simulink model "batterpack"  (R2024b)
settings: Solver=VariableStepAuto  StartTime=0.0  StopTime=10.0  RelTol=1e-3
libraries: spsParallelRLCBranchLib x432, spsDCVoltageSourceLib x144, spsIdealSwitchLib x14, spsTriangleGeneratorLib x1, spspowerguiLib x1
settings Model: Creator=32635  LastModifiedBy=32635

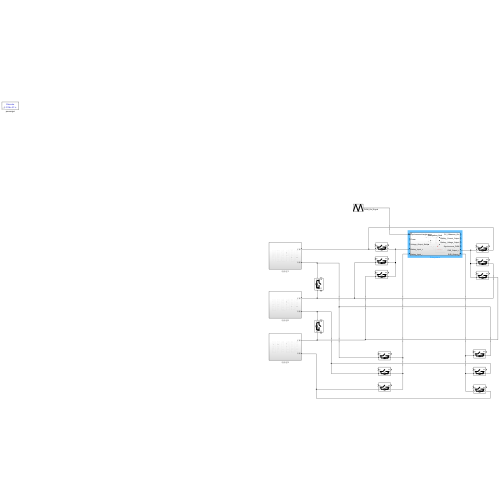
[thumbnail: Simulink's stored preview of the top-level diagram]
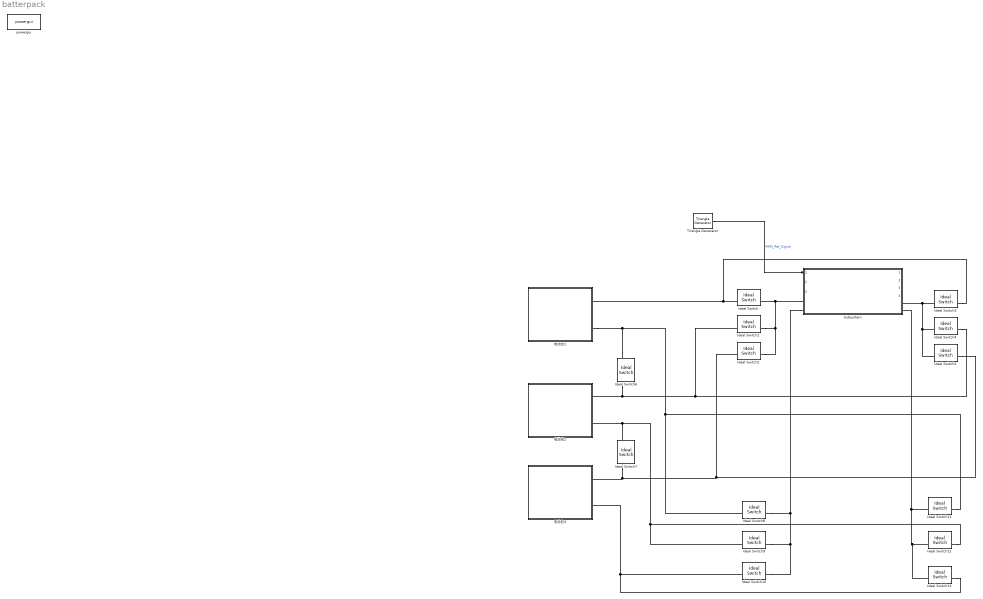
== system batterpack ==
  Ideal Switch{,1..13} (14 alike) : spsIdealSwitchLib/Ideal Switch  Ron=0.001  Lon=0  IC=0  Rs=1e5  Cs=inf  Measurements=on
  Subsystem : Subsystem  ReferencedSubsystem=Subsystem_final
  Triangle Generator : spsTriangleGeneratorLib/Triangle Generator  Freq=50000  Phase=0  Ts=0
  powergui : spspowerguiLib/powergui  Priority=1  SimulationMode=Discrete  SampleTime=1/5e4/60  frequency=60  Iterations=50  frequencyindice=0  Pbase=100e6  ErrMax=1e-4  UnitsV=kV  UnitsW=MW  buscounter=0  FunctionMessages=off  echomessages=off  EnableUseOfTLC=off  CurrentSourceSwitches=off  DisableSnubberDevices=off  DisableRonSwitches=off  DisableVfSwitches=off  DisplayEquations=off  AutomaticDiscreteSolvers=off  SolverType=Tustin/Backward Euler (TBE)  Interpol=off  ExternalGateDelay=off  methode=off  Ts=100  x0status=blocks  SPID=on  SwTol=0  HookPort=off  NonlinearTolerance=1e-4  nMaxIteration=100  ContinueOnMaxIteration=off  RestoreLinks=warning  ResistiveCurrentMeasurement=off  Frange=[0:2:500]  Ylog=off  Xlog=on  ShowGrid=off  save=off  variable=ZData  structure=0  ZoomFFT=on  StartTime=0.0  cycles=1  DisplayStyle=1  fundamental=60  FreqAxis=off  MaxFrequency=1000  frequencyindicesteady=1  RmsSteady=1  display=off
  电池包1 : Subsystem
  电池包2 : Subsystem
  电池包3 : Subsystem
  wires:
  Triangle Generator/1 -> Subsystem/1  "PWM_Ref_Signal"
  connections:
  Ideal Switch2/LConn1 -- Ideal Switch5/RConn1 -- 电池包3/RConn1 -- Ideal Switch7/RConn1
  Ideal Switch1/LConn1 -- Ideal Switch4/RConn1 -- Ideal Switch6/RConn1 -- 电池包2/RConn1
  Subsystem/LConn1 -- Ideal Switch2/RConn1 -- Ideal Switch1/RConn1 -- Ideal Switch/RConn1
  Ideal Switch/LConn1 -- Ideal Switch3/RConn1 -- 电池包1/RConn1
  Ideal Switch7/LConn1 -- Ideal Switch12/RConn1 -- Ideal Switch9/LConn1 -- 电池包2/RConn2
  Ideal Switch3/LConn1 -- Ideal Switch4/LConn1 -- Ideal Switch5/LConn1 -- Subsystem/RConn1
  电池包1/RConn2 -- Ideal Switch11/RConn1 -- Ideal Switch8/LConn1 -- Ideal Switch6/LConn1
  Ideal Switch8/RConn1 -- Ideal Switch10/RConn1 -- Ideal Switch9/RConn1 -- Subsystem/LConn2
  Ideal Switch10/LConn1 -- 电池包3/RConn2 -- Ideal Switch13/RConn1
  Ideal Switch11/LConn1 -- Ideal Switch13/LConn1 -- Ideal Switch12/LConn1 -- Subsystem/RConn2

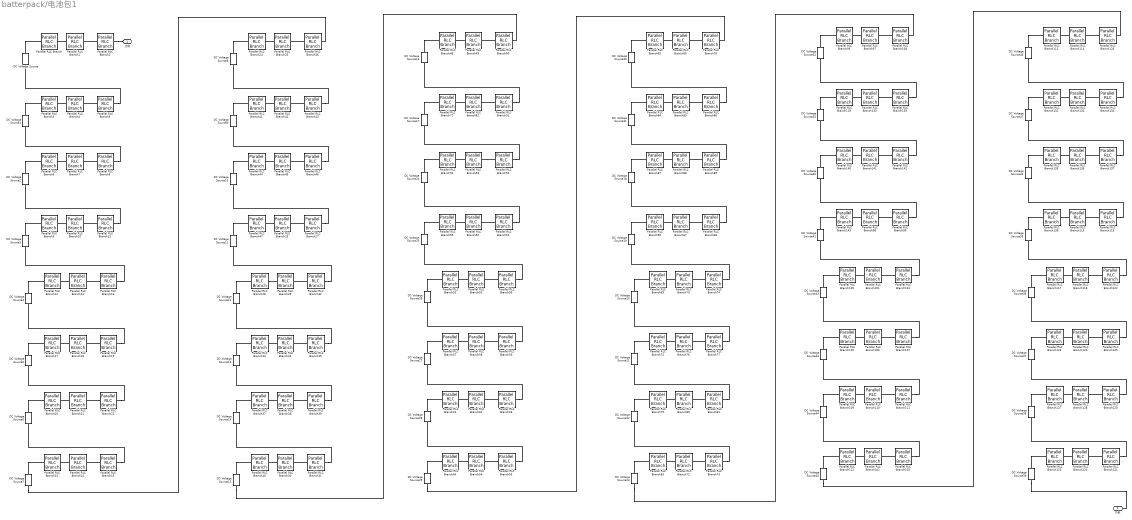
== system batterpack/电池包1 ==
  DC Voltage Source{,1..47} (48 alike) : spsDCVoltageSourceLib/DC Voltage Source  Amplitude=100  Measurements=None
  Parallel RLC Branch{,3,6,9,12,17,20,23..24,28,33,37,40..41,44,47..48,52,57,61,64..65,69,71,75,79,83..84,87,90,92,95..96,100,105,109,112..113,117,119,123,127,131..132,135,138,140,143} (48 alike) : spsParallelRLCBranchLib/Parallel RLC Branch  LConnTagsString=a  RConnTagsString=__new0  BranchType=R  Resistance=1  Inductance=1e-3  SetiL0=off  InitialCurrent=0  Capacitance=1e-6  Setx0=off  InitialVoltage=0  Measurements=None
  Parallel RLC Branch{1..2,4..5,7..8,10..11,13..16,18..19,21..22,25..27,29..32,34..36,38..39,42..43,45..46,49..51,53..56,58..60,62..63,66..68,70,72..74,76..78,80..82,85..86,88..89,91,93..94,97..99,101..104,106..108,110..111,114..116,118,120..122,124..126,128..130,133..134,136..137,139,141..142} (96 alike) : spsParallelRLCBranchLib/Parallel RLC Branch  LConnTagsString=a  RConnTagsString=__new0  BranchType=RC  Resistance=1  Inductance=1e-3  SetiL0=off  InitialCurrent=0  Capacitance=1e-6  Setx0=off  InitialVoltage=0  Measurements=None
  正极 : PMIOPort  Side=Right
  负极 : PMIOPort  Port=2  Side=Right
  connections:
  Parallel RLC Branch81/RConn1 -- DC Voltage Source21/LConn1
  Parallel RLC Branch48/LConn1 -- DC Voltage Source16/RConn1
  Parallel RLC Branch1/LConn1 -- Parallel RLC Branch/RConn1
  Parallel RLC Branch45/LConn1 -- Parallel RLC Branch44/RConn1
  Parallel RLC Branch129/RConn1 -- DC Voltage Source37/LConn1
  Parallel RLC Branch143/LConn1 -- DC Voltage Source41/RConn1
  Parallel RLC Branch8/RConn1 -- DC Voltage Source1/LConn1
  Parallel RLC Branch133/LConn1 -- Parallel RLC Branch132/RConn1
  Parallel RLC Branch87/LConn1 -- DC Voltage Source18/RConn1
  Parallel RLC Branch86/RConn1 -- DC Voltage Source30/LConn1
  Parallel RLC Branch123/LConn1 -- DC Voltage Source37/RConn1
  Parallel RLC Branch32/LConn1 -- Parallel RLC Branch29/RConn1
  Parallel RLC Branch44/LConn1 -- DC Voltage Source10/RConn1
  Parallel RLC Branch10/LConn1 -- Parallel RLC Branch9/RConn1
  DC Voltage Source15/LConn1 -- Parallel RLC Branch60/RConn1
  Parallel RLC Branch4/LConn1 -- Parallel RLC Branch3/RConn1
  Parallel RLC Branch74/RConn1 -- DC Voltage Source19/LConn1
  Parallel RLC Branch24/LConn1 -- DC Voltage Source8/RConn1
  Parallel RLC Branch107/RConn1 -- DC Voltage Source42/LConn1
  Parallel RLC Branch139/RConn1 -- DC Voltage Source32/LConn1
  Parallel RLC Branch39/LConn1 -- Parallel RLC Branch38/RConn1
  Parallel RLC Branch137/LConn1 -- Parallel RLC Branch136/RConn1
  Parallel RLC Branch126/LConn1 -- Parallel RLC Branch114/RConn1
  Parallel RLC Branch91/RConn1 -- DC Voltage Source16/LConn1
  DC Voltage Source29/LConn1 -- Parallel RLC Branch78/RConn1
  Parallel RLC Branch42/LConn1 -- Parallel RLC Branch41/RConn1
  Parallel RLC Branch68/RConn1 -- DC Voltage Source18/LConn1
  Parallel RLC Branch136/LConn1 -- Parallel RLC Branch135/RConn1
  Parallel RLC Branch5/RConn1 -- DC Voltage Source/LConn1
  Parallel RLC Branch55/LConn1 -- Parallel RLC Branch54/RConn1
  Parallel RLC Branch22/LConn1 -- Parallel RLC Branch21/RConn1
  Parallel RLC Branch27/LConn1 -- Parallel RLC Branch26/RConn1
  DC Voltage Source23/LConn1 -- Parallel RLC Branch108/RConn1
  Parallel RLC Branch80/LConn1 -- Parallel RLC Branch79/RConn1
  Parallel RLC Branch41/LConn1 -- DC Voltage Source9/RConn1
  DC Voltage Source7/LConn1 -- Parallel RLC Branch36/RConn1
  Parallel RLC Branch139/LConn1 -- Parallel RLC Branch130/RConn1
  Parallel RLC Branch99/LConn1 -- Parallel RLC Branch98/RConn1
  Parallel RLC Branch56/LConn1 -- Parallel RLC Branch53/RConn1
  Parallel RLC Branch113/LConn1 -- DC Voltage Source46/RConn1
  Parallel RLC Branch103/RConn1 -- DC Voltage Source44/LConn1
  Parallel RLC Branch94/LConn1 -- Parallel RLC Branch93/RConn1
  Parallel RLC Branch81/LConn1 -- Parallel RLC Branch80/RConn1
  Parallel RLC Branch140/LConn1 -- DC Voltage Source40/RConn1
  Parallel RLC Branch60/LConn1 -- Parallel RLC Branch49/RConn1
  Parallel RLC Branch63/LConn1 -- Parallel RLC Branch62/RConn1
  Parallel RLC Branch29/LConn1 -- Parallel RLC Branch28/RConn1
  Parallel RLC Branch104/RConn1 -- DC Voltage Source41/LConn1
  Parallel RLC Branch142/RConn1 -- DC Voltage Source33/LConn1
  Parallel RLC Branch2/LConn1 -- Parallel RLC Branch1/RConn1
  Parallel RLC Branch114/LConn1 -- Parallel RLC Branch113/RConn1
  Parallel RLC Branch16/RConn1 -- DC Voltage Source3/LConn1
  Parallel RLC Branch116/LConn1 -- Parallel RLC Branch115/RConn1
  Parallel RLC Branch67/LConn1 -- Parallel RLC Branch90/RConn1
  Parallel RLC Branch51/LConn1 -- Parallel RLC Branch50/RConn1
  Parallel RLC Branch46/LConn1 -- Parallel RLC Branch45/RConn1
  Parallel RLC Branch121/LConn1 -- Parallel RLC Branch120/RConn1
  Parallel RLC Branch104/LConn1 -- Parallel RLC Branch101/RConn1
  Parallel RLC Branch85/LConn1 -- Parallel RLC Branch84/RConn1
  Parallel RLC Branch99/RConn1 -- DC Voltage Source40/LConn1
  Parallel RLC Branch53/LConn1 -- Parallel RLC Branch52/RConn1
  Parallel RLC Branch101/LConn1 -- Parallel RLC Branch100/RConn1
  Parallel RLC Branch47/LConn1 -- DC Voltage Source11/RConn1
  Parallel RLC Branch103/LConn1 -- Parallel RLC Branch102/RConn1
  Parallel RLC Branch125/RConn1 -- DC Voltage Source36/LConn1
  Parallel RLC Branch61/LConn1 -- DC Voltage Source28/RConn1
  Parallel RLC Branch91/LConn1 -- Parallel RLC Branch82/RConn1
  Parallel RLC Branch26/LConn1 -- Parallel RLC Branch47/RConn1
  Parallel RLC Branch124/LConn1 -- Parallel RLC Branch123/RConn1
  Parallel RLC Branch132/LConn1 -- DC Voltage Source47/RConn1
  Parallel RLC Branch64/LConn1 -- DC Voltage Source29/RConn1
  Parallel RLC Branch50/LConn1 -- Parallel RLC Branch95/RConn1
  Parallel RLC Branch35/LConn1 -- Parallel RLC Branch34/RConn1
  Parallel RLC Branch30/LConn1 -- Parallel RLC Branch40/RConn1
  Parallel RLC Branch28/LConn1 -- DC Voltage Source12/RConn1
  Parallel RLC Branch86/LConn1 -- Parallel RLC Branch85/RConn1
  Parallel RLC Branch57/LConn1 -- DC Voltage Source27/RConn1
  Parallel RLC Branch13/LConn1 -- Parallel RLC Branch12/RConn1
  Parallel RLC Branch58/LConn1 -- Parallel RLC Branch57/RConn1
  Parallel RLC Branch37/LConn1 -- DC Voltage Source14/RConn1
  Parallel RLC Branch63/RConn1 -- DC Voltage Source27/LConn1
  Parallel RLC Branch/LConn1 -- DC Voltage Source/RConn1
  Parallel RLC Branch73/LConn1 -- Parallel RLC Branch72/RConn1
  Parallel RLC Branch54/LConn1 -- Parallel RLC Branch64/RConn1
  Parallel RLC Branch77/LConn1 -- Parallel RLC Branch76/RConn1
  Parallel RLC Branch76/LConn1 -- Parallel RLC Branch75/RConn1
  Parallel RLC Branch73/RConn1 -- DC Voltage Source22/LConn1
  Parallel RLC Branch31/RConn1 -- DC Voltage Source14/LConn1
  Parallel RLC Branch112/LConn1 -- DC Voltage Source45/RConn1
  Parallel RLC Branch70/LConn1 -- Parallel RLC Branch69/RConn1
  Parallel RLC Branch15/LConn1 -- Parallel RLC Branch14/RConn1
  Parallel RLC Branch59/LConn1 -- Parallel RLC Branch58/RConn1
  Parallel RLC Branch35/RConn1 -- DC Voltage Source12/LConn1
  Parallel RLC Branch49/LConn1 -- Parallel RLC Branch48/RConn1
  Parallel RLC Branch69/LConn1 -- DC Voltage Source20/RConn1
  Parallel RLC Branch51/RConn1 -- DC Voltage Source24/LConn1
  Parallel RLC Branch134/RConn1 -- DC Voltage Source46/LConn1
  Parallel RLC Branch72/LConn1 -- Parallel RLC Branch83/RConn1
  Parallel RLC Branch55/RConn1 -- DC Voltage Source28/LConn1
  Parallel RLC Branch84/LConn1 -- DC Voltage Source31/RConn1
  Parallel RLC Branch78/LConn1 -- Parallel RLC Branch66/RConn1
  Parallel RLC Branch15/RConn1 -- DC Voltage Source6/LConn1
  Parallel RLC Branch83/LConn1 -- DC Voltage Source23/RConn1
  Parallel RLC Branch117/LConn1 -- DC Voltage Source36/RConn1
  Parallel RLC Branch74/LConn1 -- Parallel RLC Branch70/RConn1
  Parallel RLC Branch90/LConn1 -- DC Voltage Source19/RConn1
  Parallel RLC Branch89/LConn1 -- Parallel RLC Branch88/RConn1
  Parallel RLC Branch106/LConn1 -- Parallel RLC Branch105/RConn1
  Parallel RLC Branch62/LConn1 -- Parallel RLC Branch61/RConn1
  Parallel RLC Branch52/LConn1 -- DC Voltage Source26/RConn1
  Parallel RLC Branch88/LConn1 -- Parallel RLC Branch87/RConn1
  Parallel RLC Branch129/LConn1 -- Parallel RLC Branch128/RConn1
  Parallel RLC Branch96/LConn1 -- DC Voltage Source32/RConn1
  Parallel RLC Branch94/RConn1 -- DC Voltage Source17/LConn1
  Parallel RLC Branch95/LConn1 -- DC Voltage Source25/RConn1
  Parallel RLC Branch56/RConn1 -- DC Voltage Source25/LConn1
  Parallel RLC Branch92/LConn1 -- DC Voltage Source24/RConn1
  Parallel RLC Branch75/LConn1 -- DC Voltage Source21/RConn1
  Parallel RLC Branch89/RConn1 -- DC Voltage Source31/LConn1
  Parallel RLC Branch111/LConn1 -- Parallel RLC Branch110/RConn1
  Parallel RLC Branch66/LConn1 -- Parallel RLC Branch65/RConn1
  Parallel RLC Branch77/RConn1 -- DC Voltage Source20/LConn1
  Parallel RLC Branch68/LConn1 -- Parallel RLC Branch67/RConn1
  Parallel RLC Branch120/LConn1 -- Parallel RLC Branch131/RConn1
  DC Voltage Source45/LConn1 -- Parallel RLC Branch126/RConn1
  Parallel RLC Branch97/LConn1 -- Parallel RLC Branch96/RConn1
  Parallel RLC Branch36/LConn1 -- Parallel RLC Branch25/RConn1
  Parallel RLC Branch9/LConn1 -- DC Voltage Source3/RConn1
  Parallel RLC Branch93/LConn1 -- Parallel RLC Branch92/RConn1
  Parallel RLC Branch79/LConn1 -- DC Voltage Source22/RConn1
  Parallel RLC Branch65/LConn1 -- DC Voltage Source30/RConn1
  Parallel RLC Branch71/LConn1 -- DC Voltage Source17/RConn1
  Parallel RLC Branch82/LConn1 -- Parallel RLC Branch71/RConn1
  Parallel RLC Branch59/RConn1 -- DC Voltage Source26/LConn1
  Parallel RLC Branch22/RConn1 -- DC Voltage Source5/LConn1
  Parallel RLC Branch18/LConn1 -- Parallel RLC Branch17/RConn1
  Parallel RLC Branch20/LConn1 -- DC Voltage Source6/RConn1
  Parallel RLC Branch12/LConn1 -- DC Voltage Source4/RConn1
  Parallel RLC Branch19/RConn1 -- DC Voltage Source4/LConn1
  Parallel RLC Branch16/LConn1 -- Parallel RLC Branch13/RConn1
  Parallel RLC Branch23/LConn1 -- DC Voltage Source7/RConn1
  Parallel RLC Branch19/LConn1 -- Parallel RLC Branch18/RConn1
  Parallel RLC Branch14/LConn1 -- Parallel RLC Branch23/RConn1
  Parallel RLC Branch17/LConn1 -- DC Voltage Source5/RConn1
  Parallel RLC Branch138/LConn1 -- DC Voltage Source35/RConn1
  Parallel RLC Branch21/LConn1 -- Parallel RLC Branch20/RConn1
  Parallel RLC Branch25/LConn1 -- Parallel RLC Branch24/RConn1
  Parallel RLC Branch27/RConn1 -- DC Voltage Source10/LConn1
  Parallel RLC Branch33/LConn1 -- DC Voltage Source13/RConn1
  Parallel RLC Branch32/RConn1 -- DC Voltage Source11/LConn1
  Parallel RLC Branch108/LConn1 -- Parallel RLC Branch97/RConn1
  Parallel RLC Branch34/LConn1 -- Parallel RLC Branch33/RConn1
  Parallel RLC Branch43/RConn1 -- DC Voltage Source8/LConn1
  Parallel RLC Branch31/LConn1 -- Parallel RLC Branch30/RConn1
  Parallel RLC Branch46/RConn1 -- DC Voltage Source9/LConn1
  Parallel RLC Branch40/LConn1 -- DC Voltage Source15/RConn1
  Parallel RLC Branch39/RConn1 -- DC Voltage Source13/LConn1
  Parallel RLC Branch135/LConn1 -- DC Voltage Source34/RConn1
  Parallel RLC Branch110/LConn1 -- Parallel RLC Branch109/RConn1
  Parallel RLC Branch100/LConn1 -- DC Voltage Source42/RConn1
  Parallel RLC Branch43/LConn1 -- Parallel RLC Branch42/RConn1
  Parallel RLC Branch5/LConn1 -- Parallel RLC Branch4/RConn1
  Parallel RLC Branch3/LConn1 -- DC Voltage Source1/RConn1
  Parallel RLC Branch6/LConn1 -- DC Voltage Source2/RConn1
  Parallel RLC Branch11/LConn1 -- Parallel RLC Branch10/RConn1
  Parallel RLC Branch107/LConn1 -- Parallel RLC Branch106/RConn1
  Parallel RLC Branch8/LConn1 -- Parallel RLC Branch7/RConn1
  Parallel RLC Branch11/RConn1 -- DC Voltage Source2/LConn1
  Parallel RLC Branch118/LConn1 -- Parallel RLC Branch117/RConn1
  Parallel RLC Branch7/LConn1 -- Parallel RLC Branch6/RConn1
  Parallel RLC Branch38/LConn1 -- Parallel RLC Branch37/RConn1
  Parallel RLC Branch134/LConn1 -- Parallel RLC Branch133/RConn1
  Parallel RLC Branch119/LConn1 -- DC Voltage Source33/RConn1
  Parallel RLC Branch142/LConn1 -- Parallel RLC Branch141/RConn1
  Parallel RLC Branch130/LConn1 -- Parallel RLC Branch119/RConn1
  Parallel RLC Branch131/LConn1 -- DC Voltage Source39/RConn1
  Parallel RLC Branch105/LConn1 -- DC Voltage Source43/RConn1
  Parallel RLC Branch127/LConn1 -- DC Voltage Source38/RConn1
  Parallel RLC Branch122/LConn1 -- Parallel RLC Branch118/RConn1
  Parallel RLC Branch116/RConn1 -- DC Voltage Source34/LConn1
  Parallel RLC Branch122/RConn1 -- DC Voltage Source35/LConn1
  Parallel RLC Branch98/LConn1 -- Parallel RLC Branch143/RConn1
  Parallel RLC Branch128/LConn1 -- Parallel RLC Branch127/RConn1
  Parallel RLC Branch115/LConn1 -- Parallel RLC Branch138/RConn1
  Parallel RLC Branch121/RConn1 -- DC Voltage Source38/LConn1
  Parallel RLC Branch109/LConn1 -- DC Voltage Source44/RConn1
  Parallel RLC Branch141/LConn1 -- Parallel RLC Branch140/RConn1
  Parallel RLC Branch137/RConn1 -- DC Voltage Source47/LConn1
  Parallel RLC Branch102/LConn1 -- Parallel RLC Branch112/RConn1
  Parallel RLC Branch111/RConn1 -- DC Voltage Source43/LConn1
  Parallel RLC Branch125/LConn1 -- Parallel RLC Branch124/RConn1
  DC Voltage Source39/LConn1 -- 负极/RConn1
  Parallel RLC Branch2/RConn1 -- 正极/RConn1

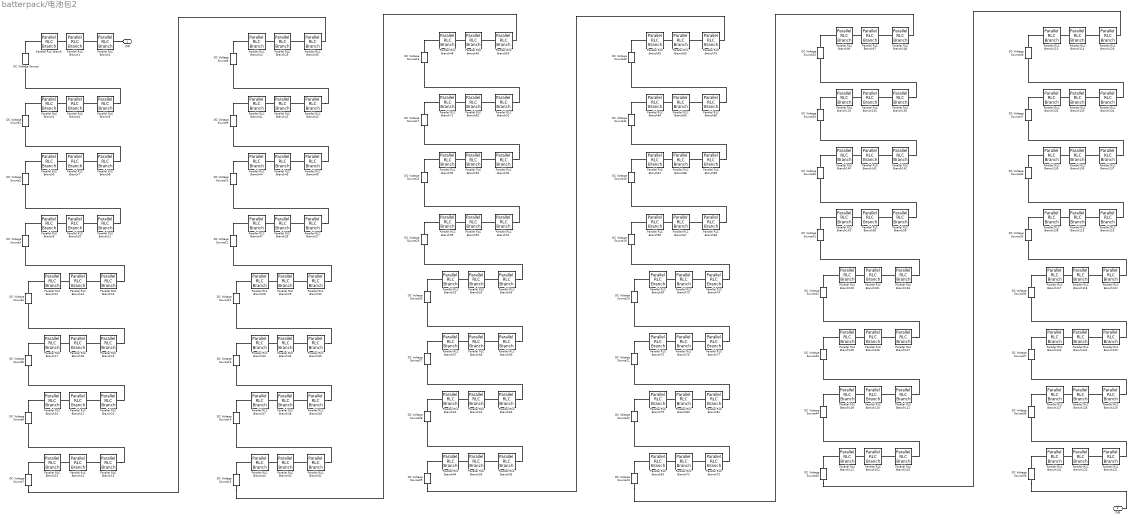
== system batterpack/电池包2 ==
  DC Voltage Source{,1..47} (48 alike) : spsDCVoltageSourceLib/DC Voltage Source  Amplitude=100  Measurements=None
  Parallel RLC Branch{,3,6,9,12,17,20,23..24,28,33,37,40..41,44,47..48,52,57,61,64..65,69,71,75,79,83..84,87,90,92,95..96,100,105,109,112..113,117,119,123,127,131..132,135,138,140,143} (48 alike) : spsParallelRLCBranchLib/Parallel RLC Branch  LConnTagsString=a  RConnTagsString=__new0  BranchType=R  Resistance=1  Inductance=1e-3  SetiL0=off  InitialCurrent=0  Capacitance=1e-6  Setx0=off  InitialVoltage=0  Measurements=None
  Parallel RLC Branch{1..2,4..5,7..8,10..11,13..16,18..19,21..22,25..27,29..32,34..36,38..39,42..43,45..46,49..51,53..56,58..60,62..63,66..68,70,72..74,76..78,80..82,85..86,88..89,91,93..94,97..99,101..104,106..108,110..111,114..116,118,120..122,124..126,128..130,133..134,136..137,139,141..142} (96 alike) : spsParallelRLCBranchLib/Parallel RLC Branch  LConnTagsString=a  RConnTagsString=__new0  BranchType=RC  Resistance=1  Inductance=1e-3  SetiL0=off  InitialCurrent=0  Capacitance=1e-6  Setx0=off  InitialVoltage=0  Measurements=None
  正极 : PMIOPort  Side=Right
  负极 : PMIOPort  Port=2  Side=Right
  connections:
  Parallel RLC Branch2/RConn1 -- 正极/RConn1
  DC Voltage Source39/LConn1 -- 负极/RConn1
  Parallel RLC Branch125/LConn1 -- Parallel RLC Branch124/RConn1
  Parallel RLC Branch111/RConn1 -- DC Voltage Source43/LConn1
  Parallel RLC Branch102/LConn1 -- Parallel RLC Branch112/RConn1
  Parallel RLC Branch137/RConn1 -- DC Voltage Source47/LConn1
  Parallel RLC Branch141/LConn1 -- Parallel RLC Branch140/RConn1
  Parallel RLC Branch109/LConn1 -- DC Voltage Source44/RConn1
  Parallel RLC Branch121/RConn1 -- DC Voltage Source38/LConn1
  Parallel RLC Branch115/LConn1 -- Parallel RLC Branch138/RConn1
  Parallel RLC Branch128/LConn1 -- Parallel RLC Branch127/RConn1
  Parallel RLC Branch98/LConn1 -- Parallel RLC Branch143/RConn1
  Parallel RLC Branch122/RConn1 -- DC Voltage Source35/LConn1
  Parallel RLC Branch116/RConn1 -- DC Voltage Source34/LConn1
  Parallel RLC Branch122/LConn1 -- Parallel RLC Branch118/RConn1
  Parallel RLC Branch127/LConn1 -- DC Voltage Source38/RConn1
  Parallel RLC Branch105/LConn1 -- DC Voltage Source43/RConn1
  Parallel RLC Branch131/LConn1 -- DC Voltage Source39/RConn1
  Parallel RLC Branch130/LConn1 -- Parallel RLC Branch119/RConn1
  Parallel RLC Branch142/LConn1 -- Parallel RLC Branch141/RConn1
  Parallel RLC Branch119/LConn1 -- DC Voltage Source33/RConn1
  Parallel RLC Branch134/LConn1 -- Parallel RLC Branch133/RConn1
  Parallel RLC Branch38/LConn1 -- Parallel RLC Branch37/RConn1
  Parallel RLC Branch7/LConn1 -- Parallel RLC Branch6/RConn1
  Parallel RLC Branch118/LConn1 -- Parallel RLC Branch117/RConn1
  Parallel RLC Branch11/RConn1 -- DC Voltage Source2/LConn1
  Parallel RLC Branch8/LConn1 -- Parallel RLC Branch7/RConn1
  Parallel RLC Branch107/LConn1 -- Parallel RLC Branch106/RConn1
  Parallel RLC Branch11/LConn1 -- Parallel RLC Branch10/RConn1
  Parallel RLC Branch6/LConn1 -- DC Voltage Source2/RConn1
  Parallel RLC Branch3/LConn1 -- DC Voltage Source1/RConn1
  Parallel RLC Branch5/LConn1 -- Parallel RLC Branch4/RConn1
  Parallel RLC Branch43/LConn1 -- Parallel RLC Branch42/RConn1
  Parallel RLC Branch100/LConn1 -- DC Voltage Source42/RConn1
  Parallel RLC Branch110/LConn1 -- Parallel RLC Branch109/RConn1
  Parallel RLC Branch135/LConn1 -- DC Voltage Source34/RConn1
  Parallel RLC Branch39/RConn1 -- DC Voltage Source13/LConn1
  Parallel RLC Branch40/LConn1 -- DC Voltage Source15/RConn1
  Parallel RLC Branch46/RConn1 -- DC Voltage Source9/LConn1
  Parallel RLC Branch31/LConn1 -- Parallel RLC Branch30/RConn1
  Parallel RLC Branch43/RConn1 -- DC Voltage Source8/LConn1
  Parallel RLC Branch34/LConn1 -- Parallel RLC Branch33/RConn1
  Parallel RLC Branch108/LConn1 -- Parallel RLC Branch97/RConn1
  Parallel RLC Branch32/RConn1 -- DC Voltage Source11/LConn1
  Parallel RLC Branch33/LConn1 -- DC Voltage Source13/RConn1
  Parallel RLC Branch27/RConn1 -- DC Voltage Source10/LConn1
  Parallel RLC Branch25/LConn1 -- Parallel RLC Branch24/RConn1
  Parallel RLC Branch21/LConn1 -- Parallel RLC Branch20/RConn1
  Parallel RLC Branch138/LConn1 -- DC Voltage Source35/RConn1
  Parallel RLC Branch17/LConn1 -- DC Voltage Source5/RConn1
  Parallel RLC Branch14/LConn1 -- Parallel RLC Branch23/RConn1
  Parallel RLC Branch19/LConn1 -- Parallel RLC Branch18/RConn1
  Parallel RLC Branch23/LConn1 -- DC Voltage Source7/RConn1
  Parallel RLC Branch16/LConn1 -- Parallel RLC Branch13/RConn1
  Parallel RLC Branch19/RConn1 -- DC Voltage Source4/LConn1
  Parallel RLC Branch12/LConn1 -- DC Voltage Source4/RConn1
  Parallel RLC Branch20/LConn1 -- DC Voltage Source6/RConn1
  Parallel RLC Branch18/LConn1 -- Parallel RLC Branch17/RConn1
  Parallel RLC Branch22/RConn1 -- DC Voltage Source5/LConn1
  Parallel RLC Branch59/RConn1 -- DC Voltage Source26/LConn1
  Parallel RLC Branch82/LConn1 -- Parallel RLC Branch71/RConn1
  Parallel RLC Branch71/LConn1 -- DC Voltage Source17/RConn1
  Parallel RLC Branch65/LConn1 -- DC Voltage Source30/RConn1
  Parallel RLC Branch79/LConn1 -- DC Voltage Source22/RConn1
  Parallel RLC Branch93/LConn1 -- Parallel RLC Branch92/RConn1
  Parallel RLC Branch9/LConn1 -- DC Voltage Source3/RConn1
  Parallel RLC Branch36/LConn1 -- Parallel RLC Branch25/RConn1
  Parallel RLC Branch97/LConn1 -- Parallel RLC Branch96/RConn1
  DC Voltage Source45/LConn1 -- Parallel RLC Branch126/RConn1
  Parallel RLC Branch120/LConn1 -- Parallel RLC Branch131/RConn1
  Parallel RLC Branch68/LConn1 -- Parallel RLC Branch67/RConn1
  Parallel RLC Branch77/RConn1 -- DC Voltage Source20/LConn1
  Parallel RLC Branch66/LConn1 -- Parallel RLC Branch65/RConn1
  Parallel RLC Branch111/LConn1 -- Parallel RLC Branch110/RConn1
  Parallel RLC Branch89/RConn1 -- DC Voltage Source31/LConn1
  Parallel RLC Branch75/LConn1 -- DC Voltage Source21/RConn1
  Parallel RLC Branch92/LConn1 -- DC Voltage Source24/RConn1
  Parallel RLC Branch56/RConn1 -- DC Voltage Source25/LConn1
  Parallel RLC Branch95/LConn1 -- DC Voltage Source25/RConn1
  Parallel RLC Branch94/RConn1 -- DC Voltage Source17/LConn1
  Parallel RLC Branch96/LConn1 -- DC Voltage Source32/RConn1
  Parallel RLC Branch129/LConn1 -- Parallel RLC Branch128/RConn1
  Parallel RLC Branch88/LConn1 -- Parallel RLC Branch87/RConn1
  Parallel RLC Branch52/LConn1 -- DC Voltage Source26/RConn1
  Parallel RLC Branch62/LConn1 -- Parallel RLC Branch61/RConn1
  Parallel RLC Branch106/LConn1 -- Parallel RLC Branch105/RConn1
  Parallel RLC Branch89/LConn1 -- Parallel RLC Branch88/RConn1
  Parallel RLC Branch90/LConn1 -- DC Voltage Source19/RConn1
  Parallel RLC Branch74/LConn1 -- Parallel RLC Branch70/RConn1
  Parallel RLC Branch117/LConn1 -- DC Voltage Source36/RConn1
  Parallel RLC Branch83/LConn1 -- DC Voltage Source23/RConn1
  Parallel RLC Branch15/RConn1 -- DC Voltage Source6/LConn1
  Parallel RLC Branch78/LConn1 -- Parallel RLC Branch66/RConn1
  Parallel RLC Branch84/LConn1 -- DC Voltage Source31/RConn1
  Parallel RLC Branch55/RConn1 -- DC Voltage Source28/LConn1
  Parallel RLC Branch72/LConn1 -- Parallel RLC Branch83/RConn1
  Parallel RLC Branch134/RConn1 -- DC Voltage Source46/LConn1
  Parallel RLC Branch51/RConn1 -- DC Voltage Source24/LConn1
  Parallel RLC Branch69/LConn1 -- DC Voltage Source20/RConn1
  Parallel RLC Branch49/LConn1 -- Parallel RLC Branch48/RConn1
  Parallel RLC Branch35/RConn1 -- DC Voltage Source12/LConn1
  Parallel RLC Branch59/LConn1 -- Parallel RLC Branch58/RConn1
  Parallel RLC Branch15/LConn1 -- Parallel RLC Branch14/RConn1
  Parallel RLC Branch70/LConn1 -- Parallel RLC Branch69/RConn1
  Parallel RLC Branch112/LConn1 -- DC Voltage Source45/RConn1
  Parallel RLC Branch31/RConn1 -- DC Voltage Source14/LConn1
  Parallel RLC Branch73/RConn1 -- DC Voltage Source22/LConn1
  Parallel RLC Branch76/LConn1 -- Parallel RLC Branch75/RConn1
  Parallel RLC Branch77/LConn1 -- Parallel RLC Branch76/RConn1
  Parallel RLC Branch54/LConn1 -- Parallel RLC Branch64/RConn1
  Parallel RLC Branch73/LConn1 -- Parallel RLC Branch72/RConn1
  Parallel RLC Branch/LConn1 -- DC Voltage Source/RConn1
  Parallel RLC Branch63/RConn1 -- DC Voltage Source27/LConn1
  Parallel RLC Branch37/LConn1 -- DC Voltage Source14/RConn1
  Parallel RLC Branch58/LConn1 -- Parallel RLC Branch57/RConn1
  Parallel RLC Branch13/LConn1 -- Parallel RLC Branch12/RConn1
  Parallel RLC Branch57/LConn1 -- DC Voltage Source27/RConn1
  Parallel RLC Branch86/LConn1 -- Parallel RLC Branch85/RConn1
  Parallel RLC Branch28/LConn1 -- DC Voltage Source12/RConn1
  Parallel RLC Branch30/LConn1 -- Parallel RLC Branch40/RConn1
  Parallel RLC Branch35/LConn1 -- Parallel RLC Branch34/RConn1
  Parallel RLC Branch50/LConn1 -- Parallel RLC Branch95/RConn1
  Parallel RLC Branch64/LConn1 -- DC Voltage Source29/RConn1
  Parallel RLC Branch132/LConn1 -- DC Voltage Source47/RConn1
  Parallel RLC Branch124/LConn1 -- Parallel RLC Branch123/RConn1
  Parallel RLC Branch26/LConn1 -- Parallel RLC Branch47/RConn1
  Parallel RLC Branch91/LConn1 -- Parallel RLC Branch82/RConn1
  Parallel RLC Branch61/LConn1 -- DC Voltage Source28/RConn1
  Parallel RLC Branch125/RConn1 -- DC Voltage Source36/LConn1
  Parallel RLC Branch103/LConn1 -- Parallel RLC Branch102/RConn1
  Parallel RLC Branch47/LConn1 -- DC Voltage Source11/RConn1
  Parallel RLC Branch101/LConn1 -- Parallel RLC Branch100/RConn1
  Parallel RLC Branch53/LConn1 -- Parallel RLC Branch52/RConn1
  Parallel RLC Branch99/RConn1 -- DC Voltage Source40/LConn1
  Parallel RLC Branch85/LConn1 -- Parallel RLC Branch84/RConn1
  Parallel RLC Branch104/LConn1 -- Parallel RLC Branch101/RConn1
  Parallel RLC Branch121/LConn1 -- Parallel RLC Branch120/RConn1
  Parallel RLC Branch46/LConn1 -- Parallel RLC Branch45/RConn1
  Parallel RLC Branch51/LConn1 -- Parallel RLC Branch50/RConn1
  Parallel RLC Branch67/LConn1 -- Parallel RLC Branch90/RConn1
  Parallel RLC Branch116/LConn1 -- Parallel RLC Branch115/RConn1
  Parallel RLC Branch16/RConn1 -- DC Voltage Source3/LConn1
  Parallel RLC Branch114/LConn1 -- Parallel RLC Branch113/RConn1
  Parallel RLC Branch2/LConn1 -- Parallel RLC Branch1/RConn1
  Parallel RLC Branch142/RConn1 -- DC Voltage Source33/LConn1
  Parallel RLC Branch104/RConn1 -- DC Voltage Source41/LConn1
  Parallel RLC Branch29/LConn1 -- Parallel RLC Branch28/RConn1
  Parallel RLC Branch63/LConn1 -- Parallel RLC Branch62/RConn1
  Parallel RLC Branch60/LConn1 -- Parallel RLC Branch49/RConn1
  Parallel RLC Branch140/LConn1 -- DC Voltage Source40/RConn1
  Parallel RLC Branch81/LConn1 -- Parallel RLC Branch80/RConn1
  Parallel RLC Branch94/LConn1 -- Parallel RLC Branch93/RConn1
  Parallel RLC Branch103/RConn1 -- DC Voltage Source44/LConn1
  Parallel RLC Branch113/LConn1 -- DC Voltage Source46/RConn1
  Parallel RLC Branch56/LConn1 -- Parallel RLC Branch53/RConn1
  Parallel RLC Branch99/LConn1 -- Parallel RLC Branch98/RConn1
  Parallel RLC Branch139/LConn1 -- Parallel RLC Branch130/RConn1
  DC Voltage Source7/LConn1 -- Parallel RLC Branch36/RConn1
  Parallel RLC Branch41/LConn1 -- DC Voltage Source9/RConn1
  Parallel RLC Branch80/LConn1 -- Parallel RLC Branch79/RConn1
  DC Voltage Source23/LConn1 -- Parallel RLC Branch108/RConn1
  Parallel RLC Branch27/LConn1 -- Parallel RLC Branch26/RConn1
  Parallel RLC Branch22/LConn1 -- Parallel RLC Branch21/RConn1
  Parallel RLC Branch55/LConn1 -- Parallel RLC Branch54/RConn1
  Parallel RLC Branch5/RConn1 -- DC Voltage Source/LConn1
  Parallel RLC Branch136/LConn1 -- Parallel RLC Branch135/RConn1
  Parallel RLC Branch68/RConn1 -- DC Voltage Source18/LConn1
  Parallel RLC Branch42/LConn1 -- Parallel RLC Branch41/RConn1
  DC Voltage Source29/LConn1 -- Parallel RLC Branch78/RConn1
  Parallel RLC Branch91/RConn1 -- DC Voltage Source16/LConn1
  Parallel RLC Branch126/LConn1 -- Parallel RLC Branch114/RConn1
  Parallel RLC Branch137/LConn1 -- Parallel RLC Branch136/RConn1
  Parallel RLC Branch39/LConn1 -- Parallel RLC Branch38/RConn1
  Parallel RLC Branch139/RConn1 -- DC Voltage Source32/LConn1
  Parallel RLC Branch107/RConn1 -- DC Voltage Source42/LConn1
  Parallel RLC Branch24/LConn1 -- DC Voltage Source8/RConn1
  Parallel RLC Branch74/RConn1 -- DC Voltage Source19/LConn1
  Parallel RLC Branch4/LConn1 -- Parallel RLC Branch3/RConn1
  DC Voltage Source15/LConn1 -- Parallel RLC Branch60/RConn1
  Parallel RLC Branch10/LConn1 -- Parallel RLC Branch9/RConn1
  Parallel RLC Branch44/LConn1 -- DC Voltage Source10/RConn1
  Parallel RLC Branch32/LConn1 -- Parallel RLC Branch29/RConn1
  Parallel RLC Branch123/LConn1 -- DC Voltage Source37/RConn1
  Parallel RLC Branch86/RConn1 -- DC Voltage Source30/LConn1
  Parallel RLC Branch87/LConn1 -- DC Voltage Source18/RConn1
  Parallel RLC Branch133/LConn1 -- Parallel RLC Branch132/RConn1
  Parallel RLC Branch8/RConn1 -- DC Voltage Source1/LConn1
  Parallel RLC Branch143/LConn1 -- DC Voltage Source41/RConn1
  Parallel RLC Branch129/RConn1 -- DC Voltage Source37/LConn1
  Parallel RLC Branch45/LConn1 -- Parallel RLC Branch44/RConn1
  Parallel RLC Branch1/LConn1 -- Parallel RLC Branch/RConn1
  Parallel RLC Branch48/LConn1 -- DC Voltage Source16/RConn1
  Parallel RLC Branch81/RConn1 -- DC Voltage Source21/LConn1

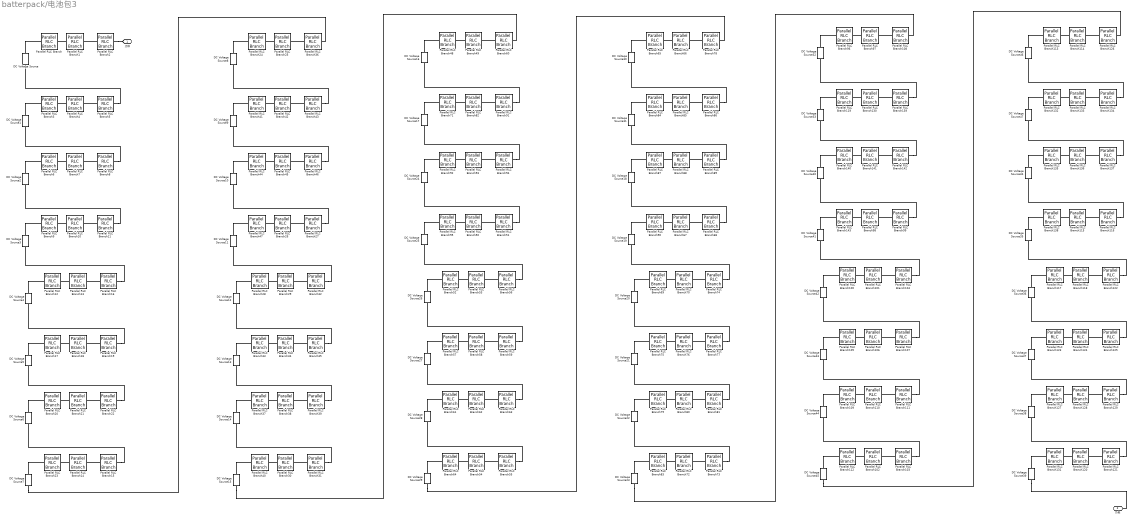
== system batterpack/电池包3 ==
  DC Voltage Source{,1..47} (48 alike) : spsDCVoltageSourceLib/DC Voltage Source  Amplitude=100  Measurements=None
  Parallel RLC Branch{,3,6,9,12,17,20,23..24,28,33,37,40..41,44,47..48,52,57,61,64..65,69,71,75,79,83..84,87,90,92,95..96,100,105,109,112..113,117,119,123,127,131..132,135,138,140,143} (48 alike) : spsParallelRLCBranchLib/Parallel RLC Branch  LConnTagsString=a  RConnTagsString=__new0  BranchType=R  Resistance=1  Inductance=1e-3  SetiL0=off  InitialCurrent=0  Capacitance=1e-6  Setx0=off  InitialVoltage=0  Measurements=None
  Parallel RLC Branch{1..2,4..5,7..8,10..11,13..16,18..19,21..22,25..27,29..32,34..36,38..39,42..43,45..46,49..51,53..56,58..60,62..63,66..68,70,72..74,76..78,80..82,85..86,88..89,91,93..94,97..99,101..104,106..108,110..111,114..116,118,120..122,124..126,128..130,133..134,136..137,139,141..142} (96 alike) : spsParallelRLCBranchLib/Parallel RLC Branch  LConnTagsString=a  RConnTagsString=__new0  BranchType=RC  Resistance=1  Inductance=1e-3  SetiL0=off  InitialCurrent=0  Capacitance=1e-6  Setx0=off  InitialVoltage=0  Measurements=None
  正极 : PMIOPort  Side=Right
  负极 : PMIOPort  Port=2  Side=Right
  connections:
  Parallel RLC Branch81/RConn1 -- DC Voltage Source21/LConn1
  Parallel RLC Branch48/LConn1 -- DC Voltage Source16/RConn1
  Parallel RLC Branch1/LConn1 -- Parallel RLC Branch/RConn1
  Parallel RLC Branch45/LConn1 -- Parallel RLC Branch44/RConn1
  Parallel RLC Branch129/RConn1 -- DC Voltage Source37/LConn1
  Parallel RLC Branch143/LConn1 -- DC Voltage Source41/RConn1
  Parallel RLC Branch8/RConn1 -- DC Voltage Source1/LConn1
  Parallel RLC Branch133/LConn1 -- Parallel RLC Branch132/RConn1
  Parallel RLC Branch87/LConn1 -- DC Voltage Source18/RConn1
  Parallel RLC Branch86/RConn1 -- DC Voltage Source30/LConn1
  Parallel RLC Branch123/LConn1 -- DC Voltage Source37/RConn1
  Parallel RLC Branch32/LConn1 -- Parallel RLC Branch29/RConn1
  Parallel RLC Branch44/LConn1 -- DC Voltage Source10/RConn1
  Parallel RLC Branch10/LConn1 -- Parallel RLC Branch9/RConn1
  DC Voltage Source15/LConn1 -- Parallel RLC Branch60/RConn1
  Parallel RLC Branch4/LConn1 -- Parallel RLC Branch3/RConn1
  Parallel RLC Branch74/RConn1 -- DC Voltage Source19/LConn1
  Parallel RLC Branch24/LConn1 -- DC Voltage Source8/RConn1
  Parallel RLC Branch107/RConn1 -- DC Voltage Source42/LConn1
  Parallel RLC Branch139/RConn1 -- DC Voltage Source32/LConn1
  Parallel RLC Branch39/LConn1 -- Parallel RLC Branch38/RConn1
  Parallel RLC Branch137/LConn1 -- Parallel RLC Branch136/RConn1
  Parallel RLC Branch126/LConn1 -- Parallel RLC Branch114/RConn1
  Parallel RLC Branch91/RConn1 -- DC Voltage Source16/LConn1
  DC Voltage Source29/LConn1 -- Parallel RLC Branch78/RConn1
  Parallel RLC Branch42/LConn1 -- Parallel RLC Branch41/RConn1
  Parallel RLC Branch68/RConn1 -- DC Voltage Source18/LConn1
  Parallel RLC Branch136/LConn1 -- Parallel RLC Branch135/RConn1
  Parallel RLC Branch5/RConn1 -- DC Voltage Source/LConn1
  Parallel RLC Branch55/LConn1 -- Parallel RLC Branch54/RConn1
  Parallel RLC Branch22/LConn1 -- Parallel RLC Branch21/RConn1
  Parallel RLC Branch27/LConn1 -- Parallel RLC Branch26/RConn1
  DC Voltage Source23/LConn1 -- Parallel RLC Branch108/RConn1
  Parallel RLC Branch80/LConn1 -- Parallel RLC Branch79/RConn1
  Parallel RLC Branch41/LConn1 -- DC Voltage Source9/RConn1
  DC Voltage Source7/LConn1 -- Parallel RLC Branch36/RConn1
  Parallel RLC Branch139/LConn1 -- Parallel RLC Branch130/RConn1
  Parallel RLC Branch99/LConn1 -- Parallel RLC Branch98/RConn1
  Parallel RLC Branch56/LConn1 -- Parallel RLC Branch53/RConn1
  Parallel RLC Branch113/LConn1 -- DC Voltage Source46/RConn1
  Parallel RLC Branch103/RConn1 -- DC Voltage Source44/LConn1
  Parallel RLC Branch94/LConn1 -- Parallel RLC Branch93/RConn1
  Parallel RLC Branch81/LConn1 -- Parallel RLC Branch80/RConn1
  Parallel RLC Branch140/LConn1 -- DC Voltage Source40/RConn1
  Parallel RLC Branch60/LConn1 -- Parallel RLC Branch49/RConn1
  Parallel RLC Branch63/LConn1 -- Parallel RLC Branch62/RConn1
  Parallel RLC Branch29/LConn1 -- Parallel RLC Branch28/RConn1
  Parallel RLC Branch104/RConn1 -- DC Voltage Source41/LConn1
  Parallel RLC Branch142/RConn1 -- DC Voltage Source33/LConn1
  Parallel RLC Branch2/LConn1 -- Parallel RLC Branch1/RConn1
  Parallel RLC Branch114/LConn1 -- Parallel RLC Branch113/RConn1
  Parallel RLC Branch16/RConn1 -- DC Voltage Source3/LConn1
  Parallel RLC Branch116/LConn1 -- Parallel RLC Branch115/RConn1
  Parallel RLC Branch67/LConn1 -- Parallel RLC Branch90/RConn1
  Parallel RLC Branch51/LConn1 -- Parallel RLC Branch50/RConn1
  Parallel RLC Branch46/LConn1 -- Parallel RLC Branch45/RConn1
  Parallel RLC Branch121/LConn1 -- Parallel RLC Branch120/RConn1
  Parallel RLC Branch104/LConn1 -- Parallel RLC Branch101/RConn1
  Parallel RLC Branch85/LConn1 -- Parallel RLC Branch84/RConn1
  Parallel RLC Branch99/RConn1 -- DC Voltage Source40/LConn1
  Parallel RLC Branch53/LConn1 -- Parallel RLC Branch52/RConn1
  Parallel RLC Branch101/LConn1 -- Parallel RLC Branch100/RConn1
  Parallel RLC Branch47/LConn1 -- DC Voltage Source11/RConn1
  Parallel RLC Branch103/LConn1 -- Parallel RLC Branch102/RConn1
  Parallel RLC Branch125/RConn1 -- DC Voltage Source36/LConn1
  Parallel RLC Branch61/LConn1 -- DC Voltage Source28/RConn1
  Parallel RLC Branch91/LConn1 -- Parallel RLC Branch82/RConn1
  Parallel RLC Branch26/LConn1 -- Parallel RLC Branch47/RConn1
  Parallel RLC Branch124/LConn1 -- Parallel RLC Branch123/RConn1
  Parallel RLC Branch132/LConn1 -- DC Voltage Source47/RConn1
  Parallel RLC Branch64/LConn1 -- DC Voltage Source29/RConn1
  Parallel RLC Branch50/LConn1 -- Parallel RLC Branch95/RConn1
  Parallel RLC Branch35/LConn1 -- Parallel RLC Branch34/RConn1
  Parallel RLC Branch30/LConn1 -- Parallel RLC Branch40/RConn1
  Parallel RLC Branch28/LConn1 -- DC Voltage Source12/RConn1
  Parallel RLC Branch86/LConn1 -- Parallel RLC Branch85/RConn1
  Parallel RLC Branch57/LConn1 -- DC Voltage Source27/RConn1
  Parallel RLC Branch13/LConn1 -- Parallel RLC Branch12/RConn1
  Parallel RLC Branch58/LConn1 -- Parallel RLC Branch57/RConn1
  Parallel RLC Branch37/LConn1 -- DC Voltage Source14/RConn1
  Parallel RLC Branch63/RConn1 -- DC Voltage Source27/LConn1
  Parallel RLC Branch/LConn1 -- DC Voltage Source/RConn1
  Parallel RLC Branch73/LConn1 -- Parallel RLC Branch72/RConn1
  Parallel RLC Branch54/LConn1 -- Parallel RLC Branch64/RConn1
  Parallel RLC Branch77/LConn1 -- Parallel RLC Branch76/RConn1
  Parallel RLC Branch76/LConn1 -- Parallel RLC Branch75/RConn1
  Parallel RLC Branch73/RConn1 -- DC Voltage Source22/LConn1
  Parallel RLC Branch31/RConn1 -- DC Voltage Source14/LConn1
  Parallel RLC Branch112/LConn1 -- DC Voltage Source45/RConn1
  Parallel RLC Branch70/LConn1 -- Parallel RLC Branch69/RConn1
  Parallel RLC Branch15/LConn1 -- Parallel RLC Branch14/RConn1
  Parallel RLC Branch59/LConn1 -- Parallel RLC Branch58/RConn1
  Parallel RLC Branch35/RConn1 -- DC Voltage Source12/LConn1
  Parallel RLC Branch49/LConn1 -- Parallel RLC Branch48/RConn1
  Parallel RLC Branch69/LConn1 -- DC Voltage Source20/RConn1
  Parallel RLC Branch51/RConn1 -- DC Voltage Source24/LConn1
  Parallel RLC Branch134/RConn1 -- DC Voltage Source46/LConn1
  Parallel RLC Branch72/LConn1 -- Parallel RLC Branch83/RConn1
  Parallel RLC Branch55/RConn1 -- DC Voltage Source28/LConn1
  Parallel RLC Branch84/LConn1 -- DC Voltage Source31/RConn1
  Parallel RLC Branch78/LConn1 -- Parallel RLC Branch66/RConn1
  Parallel RLC Branch15/RConn1 -- DC Voltage Source6/LConn1
  Parallel RLC Branch83/LConn1 -- DC Voltage Source23/RConn1
  Parallel RLC Branch117/LConn1 -- DC Voltage Source36/RConn1
  Parallel RLC Branch74/LConn1 -- Parallel RLC Branch70/RConn1
  Parallel RLC Branch90/LConn1 -- DC Voltage Source19/RConn1
  Parallel RLC Branch89/LConn1 -- Parallel RLC Branch88/RConn1
  Parallel RLC Branch106/LConn1 -- Parallel RLC Branch105/RConn1
  Parallel RLC Branch62/LConn1 -- Parallel RLC Branch61/RConn1
  Parallel RLC Branch52/LConn1 -- DC Voltage Source26/RConn1
  Parallel RLC Branch88/LConn1 -- Parallel RLC Branch87/RConn1
  Parallel RLC Branch129/LConn1 -- Parallel RLC Branch128/RConn1
  Parallel RLC Branch96/LConn1 -- DC Voltage Source32/RConn1
  Parallel RLC Branch94/RConn1 -- DC Voltage Source17/LConn1
  Parallel RLC Branch95/LConn1 -- DC Voltage Source25/RConn1
  Parallel RLC Branch56/RConn1 -- DC Voltage Source25/LConn1
  Parallel RLC Branch92/LConn1 -- DC Voltage Source24/RConn1
  Parallel RLC Branch75/LConn1 -- DC Voltage Source21/RConn1
  Parallel RLC Branch89/RConn1 -- DC Voltage Source31/LConn1
  Parallel RLC Branch111/LConn1 -- Parallel RLC Branch110/RConn1
  Parallel RLC Branch66/LConn1 -- Parallel RLC Branch65/RConn1
  Parallel RLC Branch77/RConn1 -- DC Voltage Source20/LConn1
  Parallel RLC Branch68/LConn1 -- Parallel RLC Branch67/RConn1
  Parallel RLC Branch120/LConn1 -- Parallel RLC Branch131/RConn1
  DC Voltage Source45/LConn1 -- Parallel RLC Branch126/RConn1
  Parallel RLC Branch97/LConn1 -- Parallel RLC Branch96/RConn1
  Parallel RLC Branch36/LConn1 -- Parallel RLC Branch25/RConn1
  Parallel RLC Branch9/LConn1 -- DC Voltage Source3/RConn1
  Parallel RLC Branch93/LConn1 -- Parallel RLC Branch92/RConn1
  Parallel RLC Branch79/LConn1 -- DC Voltage Source22/RConn1
  Parallel RLC Branch65/LConn1 -- DC Voltage Source30/RConn1
  Parallel RLC Branch71/LConn1 -- DC Voltage Source17/RConn1
  Parallel RLC Branch82/LConn1 -- Parallel RLC Branch71/RConn1
  Parallel RLC Branch59/RConn1 -- DC Voltage Source26/LConn1
  Parallel RLC Branch22/RConn1 -- DC Voltage Source5/LConn1
  Parallel RLC Branch18/LConn1 -- Parallel RLC Branch17/RConn1
  Parallel RLC Branch20/LConn1 -- DC Voltage Source6/RConn1
  Parallel RLC Branch12/LConn1 -- DC Voltage Source4/RConn1
  Parallel RLC Branch19/RConn1 -- DC Voltage Source4/LConn1
  Parallel RLC Branch16/LConn1 -- Parallel RLC Branch13/RConn1
  Parallel RLC Branch23/LConn1 -- DC Voltage Source7/RConn1
  Parallel RLC Branch19/LConn1 -- Parallel RLC Branch18/RConn1
  Parallel RLC Branch14/LConn1 -- Parallel RLC Branch23/RConn1
  Parallel RLC Branch17/LConn1 -- DC Voltage Source5/RConn1
  Parallel RLC Branch138/LConn1 -- DC Voltage Source35/RConn1
  Parallel RLC Branch21/LConn1 -- Parallel RLC Branch20/RConn1
  Parallel RLC Branch25/LConn1 -- Parallel RLC Branch24/RConn1
  Parallel RLC Branch27/RConn1 -- DC Voltage Source10/LConn1
  Parallel RLC Branch33/LConn1 -- DC Voltage Source13/RConn1
  Parallel RLC Branch32/RConn1 -- DC Voltage Source11/LConn1
  Parallel RLC Branch108/LConn1 -- Parallel RLC Branch97/RConn1
  Parallel RLC Branch34/LConn1 -- Parallel RLC Branch33/RConn1
  Parallel RLC Branch43/RConn1 -- DC Voltage Source8/LConn1
  Parallel RLC Branch31/LConn1 -- Parallel RLC Branch30/RConn1
  Parallel RLC Branch46/RConn1 -- DC Voltage Source9/LConn1
  Parallel RLC Branch40/LConn1 -- DC Voltage Source15/RConn1
  Parallel RLC Branch39/RConn1 -- DC Voltage Source13/LConn1
  Parallel RLC Branch135/LConn1 -- DC Voltage Source34/RConn1
  Parallel RLC Branch110/LConn1 -- Parallel RLC Branch109/RConn1
  Parallel RLC Branch100/LConn1 -- DC Voltage Source42/RConn1
  Parallel RLC Branch43/LConn1 -- Parallel RLC Branch42/RConn1
  Parallel RLC Branch5/LConn1 -- Parallel RLC Branch4/RConn1
  Parallel RLC Branch3/LConn1 -- DC Voltage Source1/RConn1
  Parallel RLC Branch6/LConn1 -- DC Voltage Source2/RConn1
  Parallel RLC Branch11/LConn1 -- Parallel RLC Branch10/RConn1
  Parallel RLC Branch107/LConn1 -- Parallel RLC Branch106/RConn1
  Parallel RLC Branch8/LConn1 -- Parallel RLC Branch7/RConn1
  Parallel RLC Branch11/RConn1 -- DC Voltage Source2/LConn1
  Parallel RLC Branch118/LConn1 -- Parallel RLC Branch117/RConn1
  Parallel RLC Branch7/LConn1 -- Parallel RLC Branch6/RConn1
  Parallel RLC Branch38/LConn1 -- Parallel RLC Branch37/RConn1
  Parallel RLC Branch134/LConn1 -- Parallel RLC Branch133/RConn1
  Parallel RLC Branch119/LConn1 -- DC Voltage Source33/RConn1
  Parallel RLC Branch142/LConn1 -- Parallel RLC Branch141/RConn1
  Parallel RLC Branch130/LConn1 -- Parallel RLC Branch119/RConn1
  Parallel RLC Branch131/LConn1 -- DC Voltage Source39/RConn1
  Parallel RLC Branch105/LConn1 -- DC Voltage Source43/RConn1
  Parallel RLC Branch127/LConn1 -- DC Voltage Source38/RConn1
  Parallel RLC Branch122/LConn1 -- Parallel RLC Branch118/RConn1
  Parallel RLC Branch116/RConn1 -- DC Voltage Source34/LConn1
  Parallel RLC Branch122/RConn1 -- DC Voltage Source35/LConn1
  Parallel RLC Branch98/LConn1 -- Parallel RLC Branch143/RConn1
  Parallel RLC Branch128/LConn1 -- Parallel RLC Branch127/RConn1
  Parallel RLC Branch115/LConn1 -- Parallel RLC Branch138/RConn1
  Parallel RLC Branch121/RConn1 -- DC Voltage Source38/LConn1
  Parallel RLC Branch109/LConn1 -- DC Voltage Source44/RConn1
  Parallel RLC Branch141/LConn1 -- Parallel RLC Branch140/RConn1
  Parallel RLC Branch137/RConn1 -- DC Voltage Source47/LConn1
  Parallel RLC Branch102/LConn1 -- Parallel RLC Branch112/RConn1
  Parallel RLC Branch111/RConn1 -- DC Voltage Source43/LConn1
  Parallel RLC Branch125/LConn1 -- Parallel RLC Branch124/RConn1
  DC Voltage Source39/LConn1 -- 负极/RConn1
  Parallel RLC Branch2/RConn1 -- 正极/RConn1
